simulink model "SimulinkTask3"  (Simulink 7.8)
settings: Solver=ode45  StartTime=0.0  StopTime=10.0  RelTol=1e-3
libraries: simulink x2
settings Model: Creator=--  LastModifiedBy=--

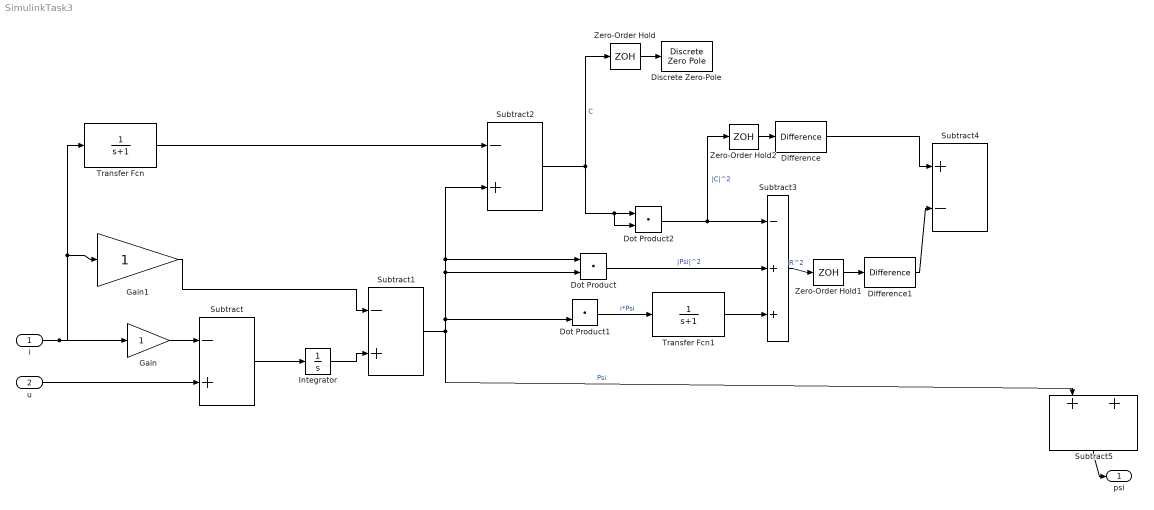
== system SimulinkTask3 ==
  i : Inport
  u : Inport  Port=2
  Difference : simulink/Discrete/Difference  ICPrevInput=0.0  InputProcessing=Inherited  OutMin=[]  OutMax=[]  OutDataType=fixdt(1, 16)  OutScaling=2^-10  DoSatur=off
  Difference1 : simulink/Discrete/Difference  ICPrevInput=0.0  InputProcessing=Inherited  OutMin=[]  OutMax=[]  OutDataType=fixdt(1, 16)  OutScaling=2^-10  DoSatur=off
  Discrete Zero-Pole : DiscreteZeroPole  Poles=[0 0.5]  Gain=1
  Dot Product : DotProduct  InputSameDT=on  OutDataTypeStr=Inherit: Inherit via internal rule
  Dot Product1 : DotProduct  InputSameDT=on  OutDataTypeStr=Inherit: Inherit via internal rule
  Dot Product2 : DotProduct  InputSameDT=on  OutDataTypeStr=Inherit: Inherit via internal rule
  Gain : Gain
  Gain1 : Gain
  Integrator : Integrator
  Subtract : Sum  Inputs=-+
  Subtract1 : Sum  Inputs=-+
  Subtract2 : Sum  Inputs=-+
  Subtract3 : Sum  Inputs=-++
  Subtract4 : Sum  Inputs=+-
  Subtract5 : Sum
  Transfer Fcn : TransferFcn  Denominator=[1 1]
  Transfer Fcn1 : TransferFcn  Denominator=[1 1]
  Zero-Order Hold : ZeroOrderHold
  Zero-Order Hold1 : ZeroOrderHold
  Zero-Order Hold2 : ZeroOrderHold
  psi : Outport
  wires:
  i/1 -> Gain1/1, Transfer Fcn/1, Gain/1
  Gain/1 -> Subtract/1
  u/1 -> Subtract/2
  Subtract/1 -> Integrator/1
  Integrator/1 -> Subtract1/2
  Gain1/1 -> Subtract1/1
  Transfer Fcn/1 -> Subtract2/1
  Subtract1/1 -> Dot Product1/2, Subtract2/2, Dot Product/1, Dot Product/2, Subtract5/1  "Psi"
  Dot Product1/1 -> Transfer Fcn1/1  "i*Psi"
  Dot Product2/1 -> Subtract3/1, Zero-Order Hold2/1  "|C|^2"
  Dot Product/1 -> Subtract3/2  "|Psi|^2"
  Transfer Fcn1/1 -> Subtract3/3
  Subtract2/1 -> Dot Product2/1, Dot Product2/2, Zero-Order Hold/1  "C"
  Subtract3/1 -> Zero-Order Hold1/1  "R^2"
  Zero-Order Hold1/1 -> Difference1/1
  Zero-Order Hold2/1 -> Difference/1
  Zero-Order Hold/1 -> Discrete Zero-Pole/1
  Difference/1 -> Subtract4/1
  Difference1/1 -> Subtract4/2
  Subtract5/1 -> psi/1
